simulink model "p2a1"  (R2023b)
settings: Solver=VariableStepAuto  StartTime=0.0  StopTime=5  RelTol=1e-3
settings Model: Creator=m96sz  LastModifiedBy=m96sz

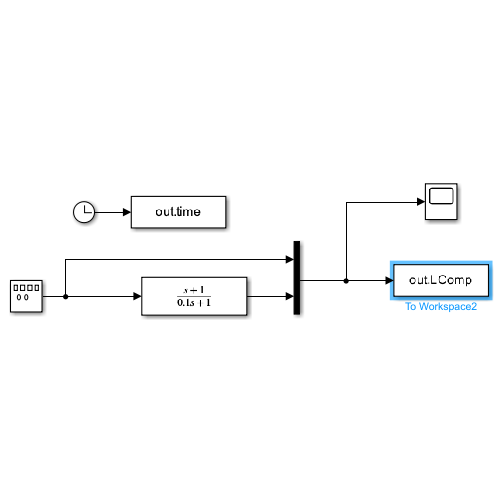
[thumbnail: Simulink's stored preview of the top-level diagram]
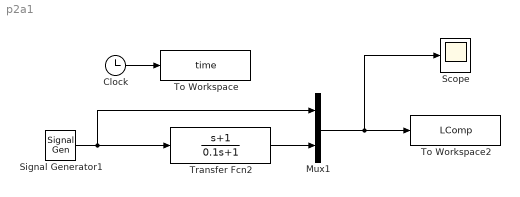
== system p2a1 ==
  Clock : Clock
      settings: Decimation=100
  Mux1 : Mux  Inputs=2
  Scope : Scope
  Signal Generator1 : SignalGenerator  WaveForm=square  Frequency=0.2
  To Workspace : ToWorkspace  VariableName=time  SampleTime=-1
  To Workspace2 : ToWorkspace  VariableName=LComp  SampleTime=-1
  Transfer Fcn2 : TransferFcn  Numerator=[1 1]  Denominator=[0.1 1]
  wires:
  Clock/1 -> To Workspace/1
  Transfer Fcn2/1 -> Mux1/2
  Signal Generator1/1 -> Transfer Fcn2/1, Mux1/1
  Mux1/1 -> To Workspace2/1, Scope/1
